simulink model "test_feedback"  (R2024b)
settings: Solver=VariableStepAuto  StartTime=0.0  StopTime=15  FixedStep=0.002  RelTol=1e-3  EnableMultiTasking=on
libraries: cstblocks x2
settings Model: ExtModeTrigDuration=10000  Creator=1163390615  LastModifiedBy=1163390615
settings SolverCC: AlgebraicLoopSolver=TrustRegion  PositivePriorityOrder=on
settings DataIOCC: ReturnWorkspaceOutputs=off
settings OptimizationCC: LifeSpan=inf
settings DebuggingCC: UnconnectedInputMsg=warning  UnconnectedOutputMsg=warning  UnconnectedLineMsg=warning  ArithmeticOperatorsInVariantConditions=warning
settings ModelReferenceCC: EnableRefExpFcnMdlSchedulingChecks=on
settings SFSimCC: SimUseLocalCustomCode=off  CustomCodeUndefinedFunction=UseInterfaceOnly
settings RTWCC: Description=QUARC Win64 Target  SystemTargetFile=quarc_win64.tlc  TemplateMakefile=quarc_default_tmf  RTWUseLocalCustomCode=off  GPUComputeCapability=3.5
settings CodeAppCC: StateflowObjectComments=on
settings STFCustomTargetCC: TargetPreCompLibLocation=C:\PROGRA~3\QUARC\lib\2016a\win64\release  TargetLangStandard=C99 (ISO)  ConcurrentExecutionCompliant=on  GRTInterface=on  SystemTargetFile=quarc_win64.tlc
settings GRTTargetCC: TargetPreCompLibLocation=C:\PROGRA~3\QUARC\lib\2016a\win64\release  ParMdlRefBuildCompliant=off  CompOptLevelCompliant=off  CombineOutputUpdateFcns=off  MatFileLogging=off  CPPClassGenCompliant=off  GRTInterface=on  UseToolchainInfoCompliant=off  ExtMode=on  ExtModeMexFile=quarc_comm
settings ConfigComp: CovMetricSettings=dswe

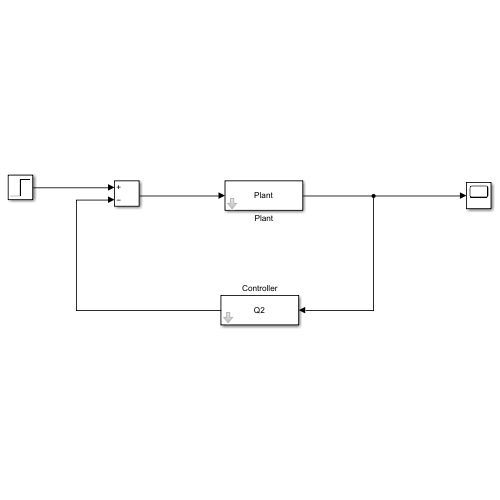
[thumbnail: Simulink's stored preview of the top-level diagram]
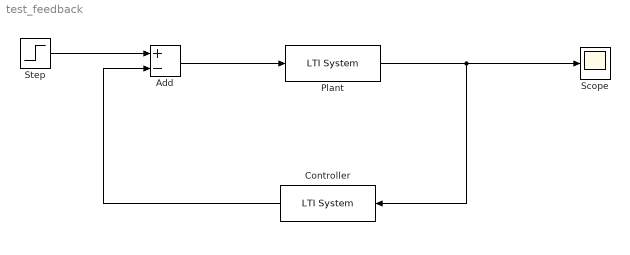
== system test_feedback ==
  Add : Sum  Inputs=+-
  Controller : cstblocks/LTI System  sys=Q2  IC=[]  PadeOrder=0
  Plant : cstblocks/LTI System  sys=Plant  IC=[]  PadeOrder=0
  Scope : Scope
  Step : Step  SampleTime=0
  wires:
  Plant/1 -> Controller/1, Scope/1
  Step/1 -> Add/1
  Controller/1 -> Add/2
  Add/1 -> Plant/1
